simulink model "nonePassFilter"  (R2016b)
settings: Solver=VariableStepAuto  StartTime=0.0  StopTime=10.0  RelTol=1e-3
settings Model: Creator=Borja Martos  LastModifiedBy=Borja Martos

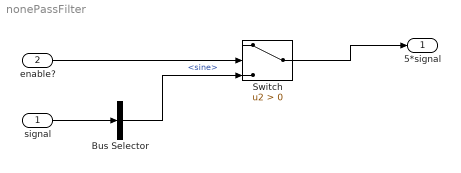
== system nonePassFilter ==
  signal : Inport  OutDataTypeStr=Bus: slBus1
  enable? : Inport  Port=2
  Bus Selector : BusSelector  OutputSignals=sine
  Switch : Switch  Criteria=u2 > Threshold
  5*signal : Outport
  wires:
  enable?/1 -> Switch/2
  signal/1 -> Bus Selector/1
  Bus Selector/1 -> Switch/3  "<sine>"
  Switch/1 -> 5*signal/1
